simulink model "exp4a"  (R2014a)
settings: Solver=ode45  StartTime=0.0  StopTime=1  RelTol=1e-3
libraries: dspsrcs4 x1
settings Model: Creator=Admin  LastModifiedBy=Admin

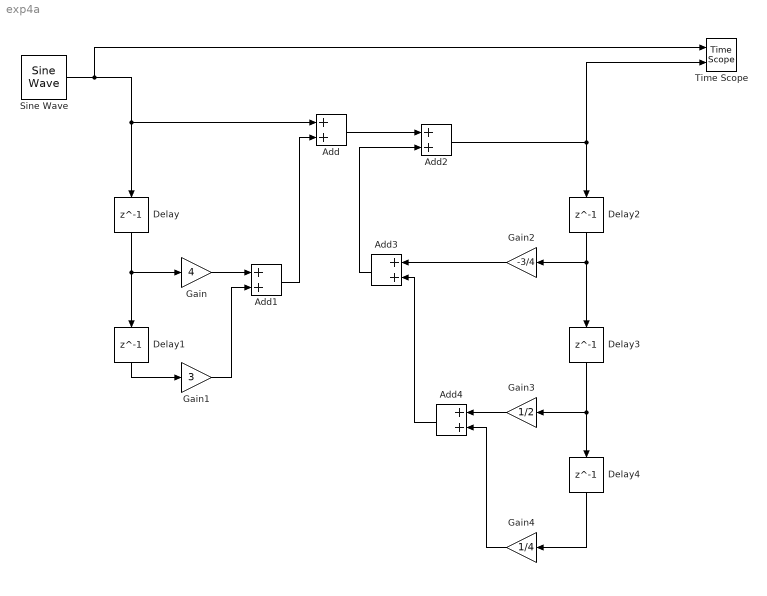
== system exp4a ==
  Add{,1..4} (5 alike) : Sum
  Delay{,1..4} (5 alike) : Delay  DelayLength=1  InitialCondition=0
  Gain : Gain  Gain=4
  Gain1 : Gain  Gain=3
  Gain2 : Gain  Gain=-3/4
  Gain3 : Gain  Gain=1/2
  Gain4 : Gain  Gain=1/4
  Sine Wave : dspsrcs4/Sine Wave  Amplitude=1  Frequency=300  Phase=0  SampleMode=Discrete  OutComplex=Real  CompMethod=Trigonometric fcn  TableSize=Speed  SampleTime=1/10000  SamplesPerFrame=1  ResetState=Restart at time zero  dataType=double  wordLen=16  udDataType=sfix(16)  fracBitsMode=Best precision  numFracBits=15  OutDataTypeStr=double  LastOutDataTypeStr=double
  Time Scope : TimeScope  NumInputPorts=2  DefaultConfigurationName=spbscopes.TimeScopeBlockCfg
  wires:
  Sine Wave/1 -> Time Scope/1, Add/1, Delay/1
  Delay/1 -> Delay1/1, Gain/1
  Delay1/1 -> Gain1/1
  Gain/1 -> Add1/1
  Add1/1 -> Add/2
  Gain1/1 -> Add1/2
  Add/1 -> Add2/1
  Add2/1 -> Delay2/1, Time Scope/2
  Delay2/1 -> Delay3/1, Gain2/1
  Delay3/1 -> Gain3/1, Delay4/1
  Delay4/1 -> Gain4/1
  Add3/1 -> Add2/2
  Gain2/1 -> Add3/1
  Gain3/1 -> Add4/1
  Gain4/1 -> Add4/2
  Add4/1 -> Add3/2
